simulink model "slack_test_simulink"  (R2023b)
settings: Solver=ode45  StartTime=0.0  StopTime=0.1  RelTol=1e-3
values from neighbouring files (symbols this model uses):
  x0 = ones(nx, 1)    [create_ocp_qp_solver_formulation.m]    (also in create_parametric_ocp_qp.m; create_pendulum_ocp.m = [0; pi; 0; 0]; create_slacked_ocp_qp_solver_formulation.m)
undefined symbols (not defined in the file or in its folder): Zl, zl, Zu, zu
settings Model: Creator=oj  LastModifiedBy=oj
settings SolverCC: AlgebraicLoopSolver=TrustRegion
settings DataIOCC: SaveFormat=StructureWithTime
settings OptimizationCC: LifeSpan=inf
settings DebuggingCC: FcnCallInpInsideContextMsg=warning  UnconnectedInputMsg=warning  UnconnectedOutputMsg=warning  UnconnectedLineMsg=warning  SFExecutionAtInitializationDiag=none  ArithmeticOperatorsInVariantConditions=warning
settings HardwareCC: ProdBitPerSizeT=32  ProdBitPerPtrDiffT=32  ProdWordSize=32  ProdHWDeviceType=Specified
settings SFSimCC: CustomCodeUndefinedFunction=UseInterfaceOnly
settings CodeAppCC: StateflowObjectComments=on

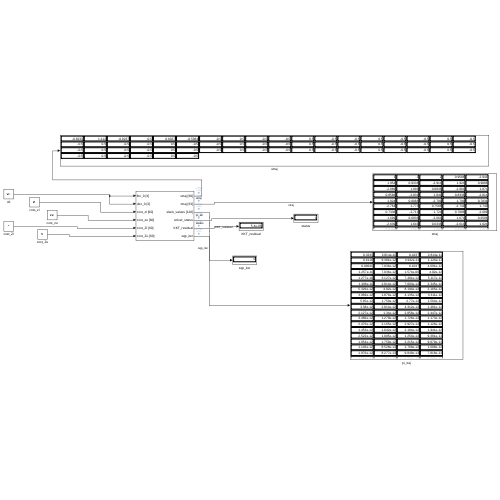
[thumbnail: Simulink's stored preview of the top-level diagram]
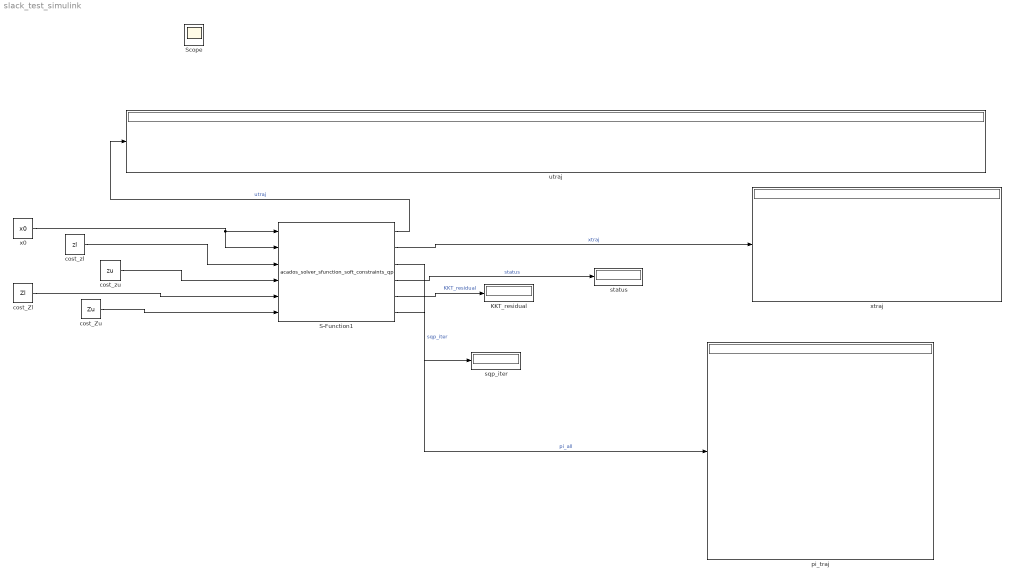
== system slack_test_simulink ==
  KKT_residual : Display
  S-Function1 : S-Function  FunctionName=acados_solver_sfunction_soft_constraints_qp  SFunctionDeploymentMode=off  EnableBusSupport=off
      mask Display:
      | global sfun_input_names sfun_output_names
      | for i = 1:length(sfun_input_names)
      | 	port_label('input', i, sfun_input_names{i})
      | end
      | for i = 1:length(sfun_output_names)
      | 	port_label('output', i, sfun_output_names{i})
      | end
  cost_Zl : Constant  Value=Zl
  cost_Zu : Constant  Value=Zu
  cost_zl : Constant  Value=zl
  cost_zu : Constant  Value=zu
  pi_traj : Display
  sqp_iter : Display
  status : Display
  utraj : Display
  x0 : Constant  Value=x0
  xtraj : Display
  Scope : Scope
  wires:
  S-Function1/5 -> KKT_residual/1  "KKT_residual"
  S-Function1/1 -> utraj/1  "utraj"
  x0/1 -> S-Function1/2, S-Function1/1
  S-Function1/2 -> xtraj/1  "xtraj"
  cost_Zu/1 -> S-Function1/6
  S-Function1/6 -> sqp_iter/1  "sqp_iter"
  S-Function1/4 -> status/1  "status"
  S-Function1/3 -> pi_traj/1  "pi_all"
  cost_Zl/1 -> S-Function1/5
  cost_zl/1 -> S-Function1/3
  cost_zu/1 -> S-Function1/4
